simulink model "etc_ctrl_mdlwork"  (R2018a)
settings: Solver=FixedStepDiscrete  StartTime=0.0  StopTime=20.0  RelTol=1e-3  EnableMultiTasking=on
model workspace (MAT data in the model file):
  Ki = 2
  Kp = 0.3
  Ts = 0.01
  e = [0; 0; 1; 1; -1; -1]
  t = [0; 2.5; 2.5; 10; 10; 20]
Description:
  | This is my help
settings Model: ParamWorkspaceSource=ReferencedWorkspace  Creator=nicholas  LastModifiedBy=bneiswan
settings DataIOCC: ExternalInput=[t, e]  LimitDataPoints=on  LoadExternalInput=on  SaveFormat=Array  SignalLoggingName=sigsOut
settings OptimizationCC: DefaultParameterBehavior=Inlined  ExpressionDepthLimit=2147483647  InitFltsAndDblsToZero=on  LifeSpan=inf
settings DebuggingCC: SaveWithParameterizedLinksMsg=none  UnderspecifiedInitializationDetection=Classic  MergeDetectMultiDrivingBlocksExec=none  MultiTaskDSMMsg=warning  MultiTaskCondExecSysMsg=none  ParameterPrecisionLossMsg=none  FcnCallInpInsideContextMsg=warning  AllowSymbolicDim=off  StateNameClashWarn=warning  SFUnexpectedBacktrackingDiag=warning  SFNoUnconditionalDefaultTransitionDiag=warning  SFExecutionAtInitializationDiag=none
settings HardwareCC: ProdBitPerPointer=32  ProdBitPerSizeT=32  ProdBitPerPtrDiffT=32  ProdLargestAtomicFloat=None  ProdIntDivRoundTo=Undefined  ProdEndianess=Unspecified  ProdWordSize=32  ProdHWDeviceType=32-bit Generic  TargetIntDivRoundTo=Zero  TargetEndianess=BigEndian  TargetHWDeviceType=Motorola PowerPC
settings ModelReferenceCC: PropagateSignalLabelsOutOfModel=off
settings CodeAppCC: StateflowObjectComments=on
settings GRTTargetCC: TargetFcnLib=ansi_tfl_tmw.mat  TargetLangStandard=C89/C90 (ANSI)  GeneratePreprocessorConditionals=Disable all  CombineOutputUpdateFcns=off  GRTInterface=on
settings ConfigComp: CovMetricSettings=dw  CovHtmlReporting=on  CovSaveCumulativeToWorkspaceVar=on  CovSaveSingleToWorkspaceVar=on  CovExternalEMLEnable=off  CovSFcnEnable=off

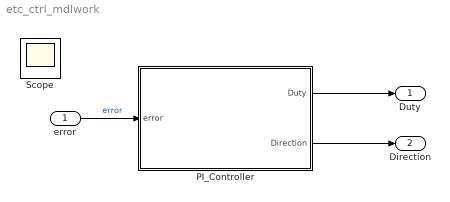
== system etc_ctrl_mdlwork ==
  error : Inport  OutDataTypeStr=double  PortDimensions=1  SampleTime=Ts
  PI_Controller : Subsystem
  Duty : Outport  OutDataTypeStr=double  PortDimensions=1  SampleTime=Ts
  Direction : Outport  Port=2  OutDataTypeStr=double  PortDimensions=1  SampleTime=Ts
  Scope : Scope
  wires:
  error/1 -> PI_Controller/1(error)  "error"
  PI_Controller/1(Duty) -> Duty/1
  PI_Controller/2(Direction) -> Direction/1

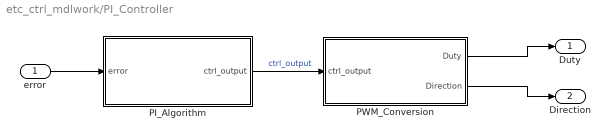
== system etc_ctrl_mdlwork/PI_Controller ==
  error : Inport
  PI_Algorithm : Subsystem
  PWM_Conversion : Subsystem
  Duty : Outport
  Direction : Outport  Port=2
  wires:
  PI_Algorithm/1(ctrl_output) -> PWM_Conversion/1(ctrl_output)  "ctrl_output"
  PWM_Conversion/2(Direction) -> Direction/1
  PWM_Conversion/1("Duty ") -> Duty/1
  error/1 -> PI_Algorithm/1(error)

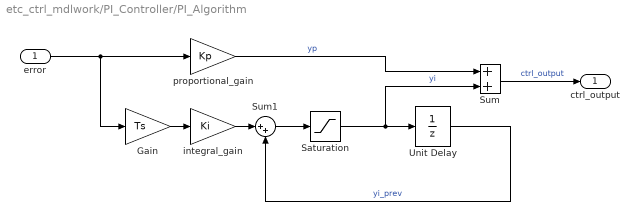
== system etc_ctrl_mdlwork/PI_Controller/PI_Algorithm ==
  error : Inport  SampleTime=Ts
      settings: AttributesFormatString=Sample time = %<SampleTime>
  Gain : Gain  Gain=Ts  SaturateOnIntegerOverflow=on  OutDataTypeStr=Inherit: Same as input  ParamDataTypeStr=Inherit: Same as input
  Saturation : Saturate  UpperLimit=1  LowerLimit=-1
      settings: AttributesFormatString=Max: %<UpperLimit>\nMin: %<LowerLimit>
  Sum : Sum  SaturateOnIntegerOverflow=on  InputSameDT=on  OutDataTypeStr=Inherit: Same as first input
  Sum1 : Sum  Inputs=|++  SaturateOnIntegerOverflow=on  InputSameDT=on  OutDataTypeStr=Inherit: Same as first input
  Unit Delay : UnitDelay  SampleTime=Ts
      settings: AttributesFormatString=yi0 = %<X0>\nSample time = %<SampleTime>
  integral_gain : Gain  Gain=Ki  SaturateOnIntegerOverflow=on  OutDataTypeStr=Inherit: Same as input  ParamDataTypeStr=Inherit: Same as input
  proportional_gain : Gain  Gain=Kp  SaturateOnIntegerOverflow=on  OutDataTypeStr=Inherit: Same as input  ParamDataTypeStr=Inherit: Same as input
  ctrl_output : Outport
  wires:
  Sum/1 -> ctrl_output/1  "ctrl_output"
  error/1 -> Gain/1, proportional_gain/1
  Saturation/1 -> Sum/2, Unit Delay/1  "yi"
  Sum1/1 -> Saturation/1
  Unit Delay/1 -> Sum1/2  "yi_prev"
  Gain/1 -> integral_gain/1
  integral_gain/1 -> Sum1/1
  proportional_gain/1 -> Sum/1  "yp"

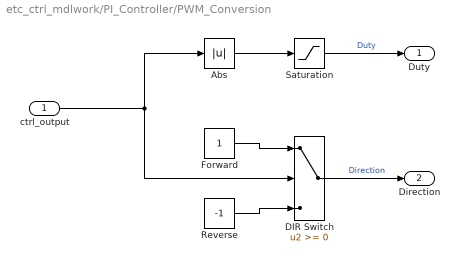
== system etc_ctrl_mdlwork/PI_Controller/PWM_Conversion ==
  ctrl_output : Inport
  Abs : Abs
  DIR Switch : Switch
      settings: AttributesFormatString=Criteria: %<Criteria>\nThreshold: %<Threshold>
  Forward : Constant  OutDataTypeStr=double
  Reverse : Constant  Value=-1  OutDataTypeStr=double
  Saturation : Saturate  UpperLimit=1  LowerLimit=0
      settings: AttributesFormatString=%<LowerLimit> < duty < %<UpperLimit>
  "Duty " : Outport
  Direction : Outport  Port=2
  wires:
  ctrl_output/1 -> Abs/1, DIR Switch/2
  Forward/1 -> DIR Switch/1
  Reverse/1 -> DIR Switch/3
  DIR Switch/1 -> Direction/1  "Direction"
  Saturation/1 -> "Duty "/1  "Duty"
  Abs/1 -> Saturation/1
